simulink model "HeatFlowDrive"  (Simulink 7.6)
settings: Solver=ode45  StartTime=0.0  StopTime="SimulTime "  RelTol=1e-3
values from neighbouring files (symbols this model uses):
  R = 25    [ParametersHeatFlow.m]
  sb = 5.67*(10^-8)    (= 5.67e-08)    [ParametersHeatFlow.m]
undefined symbols (not defined in the file or in its folder): Drive, magnitude
settings Model: Creator=conid  LastModifiedBy=conid

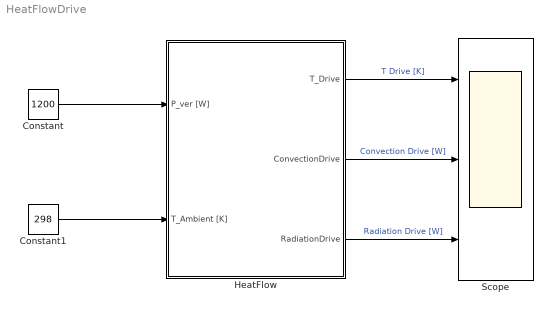
== system HeatFlowDrive ==
  Constant : Constant  Value=1200
  Constant1 : Constant  Value=298
  HeatFlow : Subsystem  TreatAsAtomicUnit=on
  Scope : Scope  NumInputPorts=3
      settings: YMin=-5~-5~-5  YMax=5~5~5  SaveName=Scp_HeatFlow
  wires:
  Constant/1 -> HeatFlow/1(P_ver [W])
  Constant1/1 -> HeatFlow/2(T_Ambient [K])
  HeatFlow/1(T_Drive) -> Scope/1  "T Drive [K]"
  HeatFlow/2(ConvectionDrive) -> Scope/2  "Convection Drive [W]"
  HeatFlow/3(RadiationDrive) -> Scope/3  "Radiation Drive [W]"

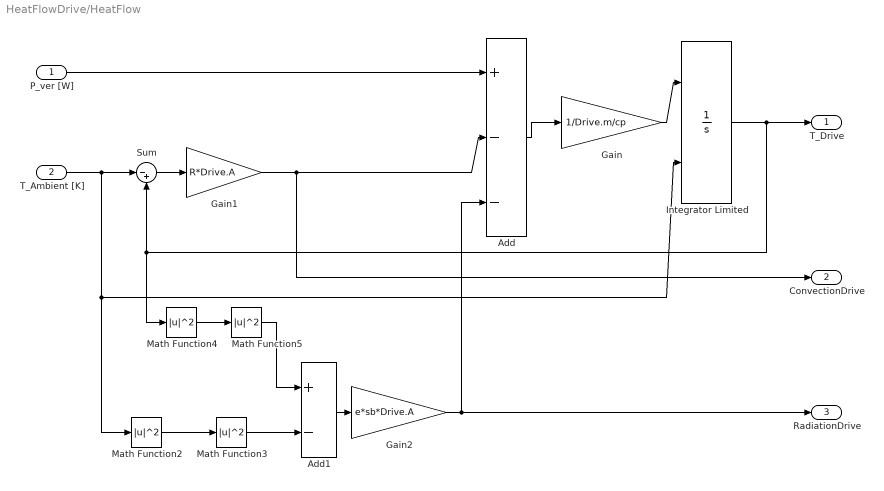
== system HeatFlowDrive/HeatFlow ==
  P_ver [W] : Inport
  T_Ambient [K] : Inport  Port=2
  Add : Sum  Inputs=+--
  Add1 : Sum  Inputs=+-
  Gain : Gain  Gain=1/Drive.m/cp
  Gain1 : Gain  Gain=R*Drive.A
  Gain2 : Gain  Gain=e*sb*Drive.A
  Integrator Limited : Integrator  InitialConditionSource=external  LimitOutput=on  ZeroCross=off
  Math Function{2..5} (4 alike) : Math  Operator=magnitude^2  SaturateOnIntegerOverflow=on
  Sum : Sum  Inputs=|-+
  T_Drive : Outport
  ConvectionDrive : Outport  Port=2
  RadiationDrive : Outport  Port=3
  wires:
  P_ver [W]/1 -> Add/1
  T_Ambient [K]/1 -> Sum/1, Integrator Limited/2, Math Function2/1
  Sum/1 -> Gain1/1
  Gain/1 -> Integrator Limited/1
  Gain1/1 -> Add/2, ConvectionDrive/1
  Integrator Limited/1 -> T_Drive/1, Sum/2, Math Function4/1
  Add/1 -> Gain/1
  Gain2/1 -> Add/3, RadiationDrive/1
  Math Function2/1 -> Math Function3/1
  Math Function4/1 -> Math Function5/1
  Math Function5/1 -> Add1/1
  Math Function3/1 -> Add1/2
  Add1/1 -> Gain2/1
